simulink model "ctrlauto_tp1_nn"  (R2018a)
settings: Solver=ode45  StartTime=0.0  StopTime=25  FixedStep=0.001  RelTol=1e-3
undefined symbols (not defined in the file or in its folder): Amd, Bmd, Cmd, DiscIntNeverNeededParam, Ki, Kp, L, Ts, u_eq, x_eq, y_eq
settings Model: Creator=aghersin  LastModifiedBy=grein

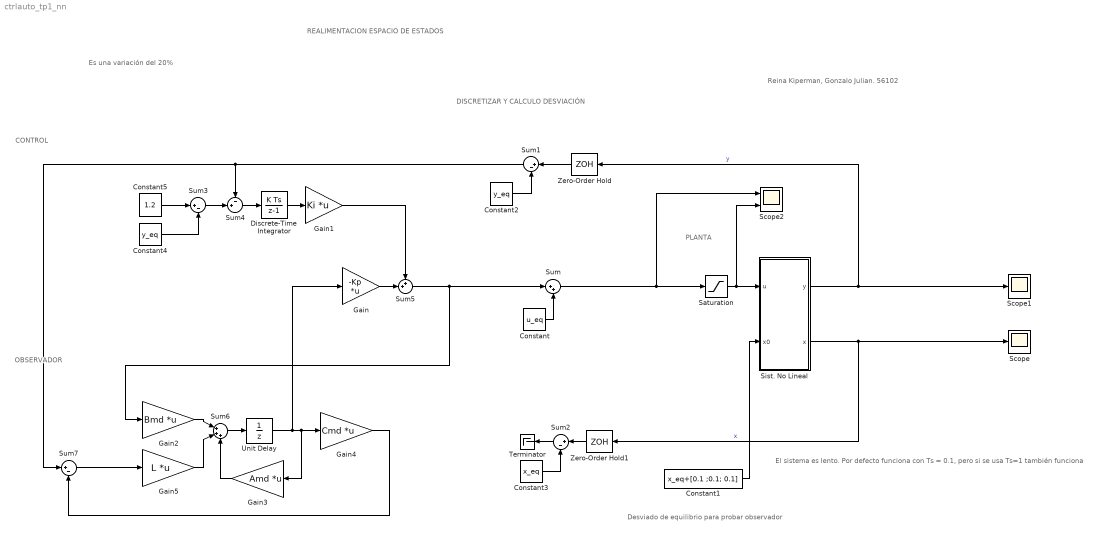
== system ctrlauto_tp1_nn ==
  note: El sistema es lento. Por defecto funciona con Ts = 0.1, pero si se usa Ts=1 también funciona
  note: Reina Kiperman, Gonzalo Julian. 56102
  note: REALIMENTACION ESPACIO DE ESTADOS
  note: Es una variación del 20%
  note: Desviado de equilibrio para probar observador
  note: OBSERVADOR
  note: DISCRETIZAR Y CALCULO DESVIACIÓN
  note: CONTROL
  note: PLANTA
  Constant : Constant  Value=u_eq
  Constant1 : Constant  Value=x_eq+[0.1 ;0.1; 0.1]
  Constant2 : Constant  Value=y_eq
  Constant3 : Constant  Value=x_eq
  Constant4 : Constant  Value=y_eq
  Constant5 : Constant  Value=1.2
  Discrete-Time Integrator : DiscreteIntegrator  SampleTime=Ts  ICPrevOutput=DiscIntNeverNeededParam  ICPrevScaledInput=DiscIntNeverNeededParam
  Gain : Gain  Gain=-Kp  Multiplication=Matrix(K*u)
  Gain1 : Gain  Gain=Ki  Multiplication=Matrix(K*u)
  Gain2 : Gain  Gain=Bmd  Multiplication=Matrix(K*u)
  Gain3 : Gain  Gain=Amd  Multiplication=Matrix(K*u)
  Gain4 : Gain  Gain=Cmd  Multiplication=Matrix(K*u)
  Gain5 : Gain  Gain=L  Multiplication=Matrix(K*u)
  Saturation : Saturate  UpperLimit=2  LowerLimit=0
  Scope : Scope
  Scope1 : Scope
  Scope2 : Scope  NumInputPorts=2
  "Sist. No Lineal " : Subsystem
  Sum : Sum  Inputs=|++
  Sum{1..3,7} (4 alike) : Sum  Inputs=|+-
  Sum4 : Sum  Inputs=-+|
  Sum5 : Sum  Inputs=++|
  Sum6 : Sum  Inputs=|+++
  Terminator : Terminator
  Unit Delay : UnitDelay  SampleTime=Ts  HasFrameUpgradeWarning=on
  Zero-Order Hold : ZeroOrderHold  SampleTime=Ts
  Zero-Order Hold1 : ZeroOrderHold  SampleTime=Ts
  wires:
  "Sist. No Lineal "/2(x) -> Zero-Order Hold1/1, Scope/1  "x"
  "Sist. No Lineal "/1(y) -> Zero-Order Hold/1, Scope1/1  "y"
  Sum/1 -> Scope2/1, Saturation/1
  Constant/1 -> Sum/2
  Constant1/1 -> "Sist. No Lineal "/2(x0)
  Constant2/1 -> Sum1/2
  Constant3/1 -> Sum2/2
  Constant5/1 -> Sum3/1
  Constant4/1 -> Sum3/2
  Sum4/1 -> Discrete-Time Integrator/1
  Discrete-Time Integrator/1 -> Gain1/1
  Sum5/1 -> Gain2/1, Sum/1
  Zero-Order Hold/1 -> Sum1/1
  Zero-Order Hold1/1 -> Sum2/1
  Sum3/1 -> Sum4/2
  Sum1/1 -> Sum7/1, Sum4/1
  Gain/1 -> Sum5/2
  Gain1/1 -> Sum5/1
  Saturation/1 -> Scope2/2, "Sist. No Lineal "/1(u)
  Sum7/1 -> Gain5/1
  Unit Delay/1 -> Gain/1, Gain4/1, Gain3/1
  Sum6/1 -> Unit Delay/1
  Gain3/1 -> Sum6/3
  Gain2/1 -> Sum6/1
  Gain5/1 -> Sum6/2
  Gain4/1 -> Sum7/2
  Sum2/1 -> Terminator/1

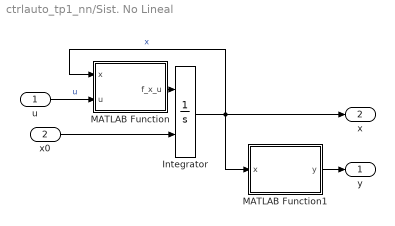
== system ctrlauto_tp1_nn/Sist. No Lineal  ==
  u : Inport
  x0 : Inport  Port=2
  Integrator : Integrator  InitialConditionSource=external
  MATLAB Function : MATLAB Function  TreatAsAtomicUnit=on
  MATLAB Function1 : MATLAB Function  TreatAsAtomicUnit=on
  y : Outport  VectorParamsAs1DForOutWhenUnconnected=off
  x : Outport  Port=2  VectorParamsAs1DForOutWhenUnconnected=off
  wires:
  u/1 -> MATLAB Function/2(u)  "u"
  MATLAB Function/1(f_x_u) -> Integrator/1
  Integrator/1 -> MATLAB Function1/1(x), x/1, MATLAB Function/1(x)  "x"
  x0/1 -> Integrator/2
  MATLAB Function1/1(y) -> y/1

== matlab function ctrlauto_tp1_nn/Sist. No Lineal /MATLAB Function ==
  data: x input; u input; f_x_u output
function f_x_u = f(x,u)

H_1 = x(1);
H_2 = x(2);
H_3 = x(3);
Q_i = u;

H_1_dot_eq = Q_i - sqrt(H_1-H_2);
H_2_dot_eq = sqrt(H_1-H_2)-sqrt(H_2-H_3);
H_3_dot_eq = sqrt(H_2-H_3)-sqrt(H_3);

f_x_u = [H_1_dot_eq ; H_2_dot_eq ; H_3_dot_eq];

== matlab function ctrlauto_tp1_nn/Sist. No Lineal /MATLAB Function1 ==
  data: x input; y output
function y = fcn(x)
    H_3 = x(3);
    y = sqrt(H_3);
